simulink model "DC_motor_with_PID"  (R2016a)
settings: Solver=VariableStepAuto  StartTime=0.0  StopTime=30  RelTol=1e-3
undefined symbols (not defined in the file or in its folder): B, J, K, L, R
libraries: simulink x1
settings Model: Creator=faiq1  LastModifiedBy=faiq1

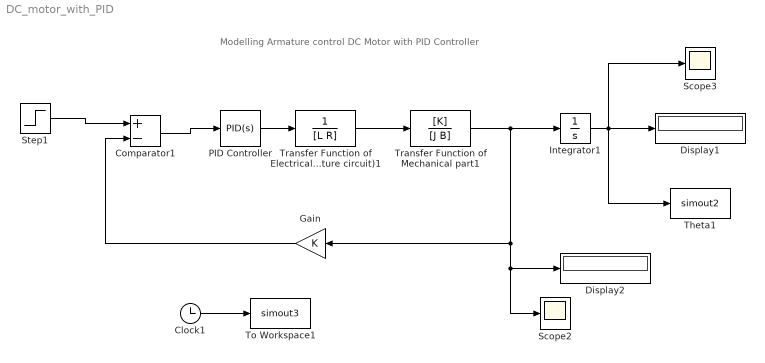
== system DC_motor_with_PID ==
  note: Modelling Armature control DC Motor
      | with PID Controller
  Clock1 : Clock
  Comparator1 : Sum  Inputs=+-
  Display1 : Display
  Display2 : Display
  Gain : Gain  Gain=K
  Integrator1 : Integrator
  PID Controller : simulink/Continuous/PID Controller  Controller=PID  TimeDomain=Continuous-time  SampleTime=-1  IntegratorMethod=Forward Euler  FilterMethod=Forward Euler  Form=Parallel  UseFilter=on  ControllerParametersSource=internal  P=5.35135484098841  I=1.56068395488721  D=2.40425569326345  N=3.71138043424136  InitialConditionSource=internal  InitialConditionForIntegrator=0  InitialConditionForFilter=0  ExternalReset=none  LimitOutput=off  UpperSaturationLimit=inf  LowerSaturationLimit=-inf  LinearizeAsGain=on  AntiWindupMode=none  Kb=1  TrackingMode=off  Kt=1  PParamMin=[]  PParamMax=[]  IParamMin=[]  IParamMax=[]  DParamMin=[]  DParamMax=[]  NParamMin=[]  NParamMax=[]  KbParamMin=[]  KbParamMax=[]  KtParamMin=[]  KtParamMax=[]  POutMin=[]  POutMax=[]  IOutMin=[]  IOutMax=[]  DOutMin=[]  DOutMax=[]  NOutMin=[]  NOutMax=[]  KbOutMin=[]  KbOutMax=[]  KtOutMin=[]  KtOutMax=[]  IntegratorOutMin=[]  IntegratorOutMax=[]  FilterOutMin=[]  FilterOutMax=[]  SumOutMin=[]  SumOutMax=[]  SumI1OutMin=[]  SumI1OutMax=[]  SumI2OutMin=[]  SumI2OutMax=[]  SumI3OutMin=[]  SumI3OutMax=[]  SumDOutMin=[]  SumDOutMax=[]  SaturationOutMin=[]  SaturationOutMax=[]  IntegratorContinuousStateAttributes=''  IntegratorStateMustResolveToSignalObject=off  IntegratorRTWStateStorageClass=Auto  FilterContinuousStateAttributes=''  FilterStateMustResolveToSignalObject=off  FilterRTWStateStorageClass=Auto  DifferentiatorICPrevScaledInput=0  DifferentiatorOutMin=[]  DifferentiatorOutMax=[]
  Scope2 : Scope
  Scope3 : Scope
  Step1 : Step  Time=0  After=14.4  SampleTime=0
  Theta1 : ToWorkspace  VariableName=simout2  SaveFormat=Timeseries  SampleTime=-1
  To Workspace1 : ToWorkspace  VariableName=simout3  SaveFormat=Timeseries  SampleTime=-1
  Transfer Function of Electrical part (Armature circuit)1 : TransferFcn  Denominator=[L R]
  Transfer Function of Mechanical part1 : TransferFcn  Numerator=[K]  Denominator=[J B]
  wires:
  Transfer Function of Electrical part (Armature circuit)1/1 -> Transfer Function of Mechanical part1/1
  Integrator1/1 -> Scope3/1, Display1/1, Theta1/1
  Clock1/1 -> To Workspace1/1
  Step1/1 -> Comparator1/1
  Gain/1 -> Comparator1/2
  Transfer Function of Mechanical part1/1 -> Integrator1/1, Gain/1, Display2/1, Scope2/1
  Comparator1/1 -> PID Controller/1
  PID Controller/1 -> Transfer Function of Electrical part (Armature circuit)1/1
